simulink model "schema_di_controllo_progetto"  (R2023b)
settings: Solver=VariableStepAuto  StartTime=0.0  StopTime=10.0  RelTol=1e-3
model workspace (MAT data in the model file):
  u_e = 74050
  x_1e = 0.5
  x_e = [0.5 0]
values from neighbouring files (symbols this model uses):
  C = [1,0]    [progetto.m]
  WW = 2    [progetto.m]
libraries: cstblocks x1
settings Model: Creator=guidocarnevale  LastModifiedBy=joseph

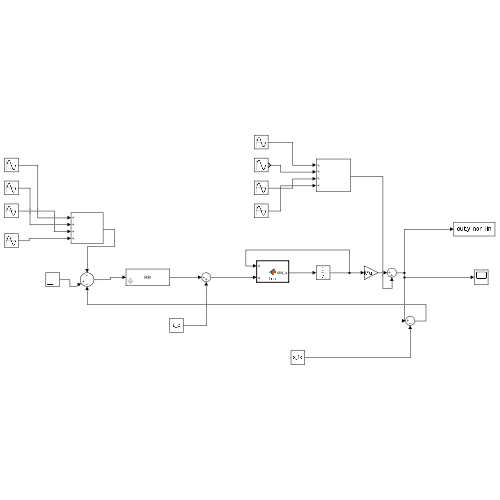
[thumbnail: Simulink's stored preview of the top-level diagram]
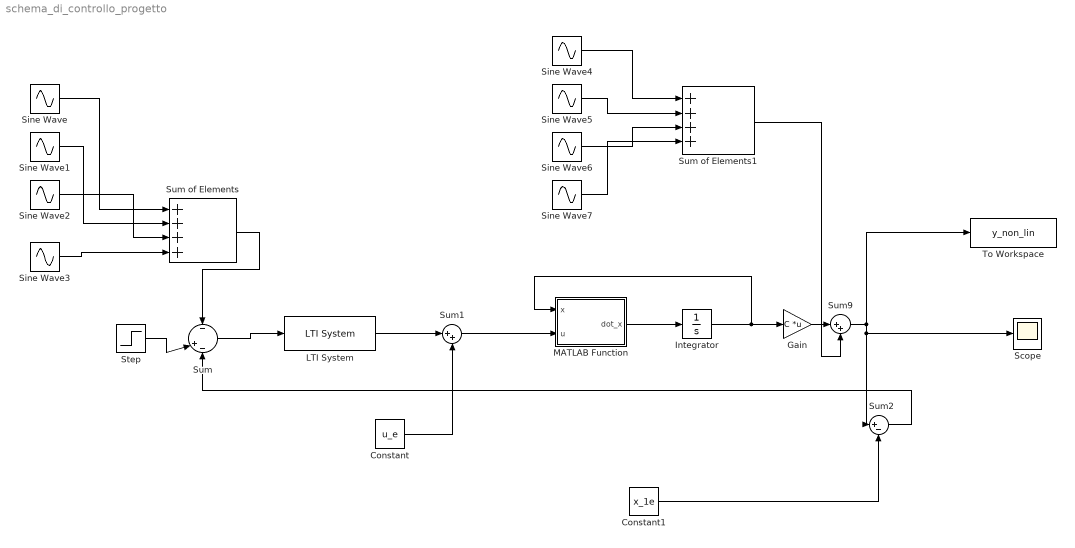
== system schema_di_controllo_progetto ==
  Constant : Constant  Value=u_e
  Constant1 : Constant  Value=x_1e
  Gain : Gain  Gain=C  Multiplication=Matrix(K*u)
  Integrator : Integrator  InitialCondition=[0.5;0]
  LTI System : cstblocks/LTI System  sys=RR  IC=[]  PadeOrder=0
  MATLAB Function : MATLAB Function  TreatAsAtomicUnit=on
  Scope : Scope
  Sine Wave : Sin  Amplitude=0.2  Frequency=5e4  SampleTime=0
  Sine Wave1 : Sin  Amplitude=0.2  Frequency=5e4*2  SampleTime=0
  Sine Wave2 : Sin  Amplitude=0.2  Frequency=5e4*3  SampleTime=0
  Sine Wave3 : Sin  Amplitude=0.2  Frequency=5e4*4  SampleTime=0
  Sine Wave4 : Sin  Amplitude=2  Frequency=0.125  SampleTime=0
  Sine Wave5 : Sin  Amplitude=2  Frequency=0.125*2  SampleTime=0
  Sine Wave6 : Sin  Amplitude=2  Frequency=0.125*3  SampleTime=0
  Sine Wave7 : Sin  Amplitude=2  Frequency=0.125*4  SampleTime=0
  Step : Step  Time=0  After=WW  SampleTime=0
  Sum : Sum  Inputs=-|+-
  Sum of Elements : Sum  Inputs=++++
  Sum of Elements1 : Sum  Inputs=++++
  Sum1 : Sum  Inputs=|++
  Sum2 : Sum  Inputs=|+-
  Sum9 : Sum  Inputs=|++
  To Workspace : ToWorkspace  VariableName=y_non_lin  SaveFormat=Timeseries  SampleTime=-1
  wires:
  MATLAB Function/1(dot_x) -> Integrator/1
  Integrator/1 -> MATLAB Function/1(x), Gain/1
  Constant/1 -> Sum1/2
  Sum1/1 -> MATLAB Function/2(u)
  Sum2/1 -> Sum/3
  Constant1/1 -> Sum2/2
  Gain/1 -> Sum9/1
  Sine Wave/1 -> Sum of Elements/1
  Sine Wave1/1 -> Sum of Elements/2
  Sine Wave2/1 -> Sum of Elements/3
  Sine Wave3/1 -> Sum of Elements/4
  Sum9/1 -> To Workspace/1, Scope/1, Sum2/1
  Sum/1 -> LTI System/1
  LTI System/1 -> Sum1/1
  Sine Wave4/1 -> Sum of Elements1/1
  Sine Wave5/1 -> Sum of Elements1/2
  Sine Wave6/1 -> Sum of Elements1/3
  Sine Wave7/1 -> Sum of Elements1/4
  Step/1 -> Sum/2
  Sum of Elements/1 -> Sum/1
  Sum of Elements1/1 -> Sum9/2

== matlab function schema_di_controllo_progetto/MATLAB Function ==
  data: x input; u input; dot_x output
function dot_x = fcn(x,u)

mm      = 5000; 
gg      = 9.81; 
kk      = 5e4;  
bb      = 250;  
beta    = 0.1;
n       = 3;


dot_x = zeros(2,1);

dot_x(1) = x(2);

dot_x(2) = - gg - bb/mm * x(2) - kk/mm*x(1) - beta/mm * (x(2)^3 +n*x(2)*(sin( n*x(2) ))^2 ) + u/mm ;
